simulink model "ModeleRobot"  (Simulink 7.4)
settings: Solver=FixedStepDiscrete  StartTime=0.0  StopTime=Inf  FixedStep=Te  RelTol=1e-3
values from neighbouring files (symbols this model uses):
  EQUIPE_JAUNE = 0    [ModeleRobot_ini.m]
  EQUIPE_VERTE = 1    [ModeleRobot_ini.m]
  JUST_HOMOLO = 1    [ModeleRobot_ini.m]
  MAX_SPEED_SERVOS = 0    [ModeleRobot_ini.m]
  PI = pi    (= 3.14159265359)    [ModeleRobot_ini.m]
  SERVO_BRAS_D = 14    [ModeleRobot_ini.m]
  SERVO_BRAS_D_FERME = 5    [ModeleRobot_ini.m]
  SERVO_BRAS_D_OUVERT = 104    [ModeleRobot_ini.m]
  SERVO_BRAS_G = 15    [ModeleRobot_ini.m]
  SERVO_BRAS_G_FERME = 18    [ModeleRobot_ini.m]
  SERVO_BRAS_G_OUVERT = 62    [ModeleRobot_ini.m]
  SERVO_INCLINAISON = 13    [ModeleRobot_ini.m]
  SERVO_INCLINAISON_DROIT = 143    [ModeleRobot_ini.m]
  SERVO_INCLINAISON_PENCHE = 24    [ModeleRobot_ini.m]
  STT = 1    [ModeleRobot_ini.m]
  Te = 0.02    [ModeleRobot_ini.m]
undefined symbols (not defined in the file or in its folder): SERVO_BEQUILLE
libraries: simulink x10
settings Model: Creator=Admin  LastModifiedBy=PC
settings DataIOCC: LimitDataPoints=off  SaveFormat=StructureWithTime
settings OptimizationCC: UseIntDivNetSlope=on  PassReuseOutputArgsAs=Individual arguments  ZeroExternalMemoryAtStartup=off  ZeroInternalMemoryAtStartup=off  EfficientFloat2IntCast=on  OptimizeModelRefInitCode=on  LifeSpan=Inf
settings DebuggingCC: SaveWithParameterizedLinksMsg=none  SignalResolutionControl=TryResolveAllWithWarning  MultiTaskDSMMsg=warning  MultiTaskCondExecSysMsg=none
settings HardwareCC: ProdIntDivRoundTo=Zero  ProdEndianess=LittleEndian  ProdHWDeviceType=Generic->32-bit x86 compatible
settings SFSimCC: SFSimEnableDebug=off  SFSimOverflowDetection=off  SFSimEcho=off  SimIntegrity=off  SimBuildMode=sf_nonincremental_build
settings RTWCC: SystemTargetFile=ert.tlc  GenCodeOnly=on  GenerateMakefile=off  TemplateMakefile=ert_default_tmf  PostCodeGenCommand=packNGo(buildInfo);  Description=Real-Time Workshop Embedded Coder  ProcessScript=ert_make_rtw_hook  IncludeERTFirstTime=on  RTWCompilerOptimization=On  CheckMdlBeforeBuild=Warning
settings CodeAppCC: IgnoreCustomStorageClasses=off
settings ERTTargetCC: UtilityFuncGeneration=Shared location  MultiwordLength=2048  IncludeMdlTerminateFcn=off  SuppressErrorStatus=on  SupportNonFinite=off  ERTCustomFileTemplate=example_file_process.tlc  GlobalDataDefinition=InSourceFile  GlobalDataReference=InSourceFile  ConvertIfToSwitch=off

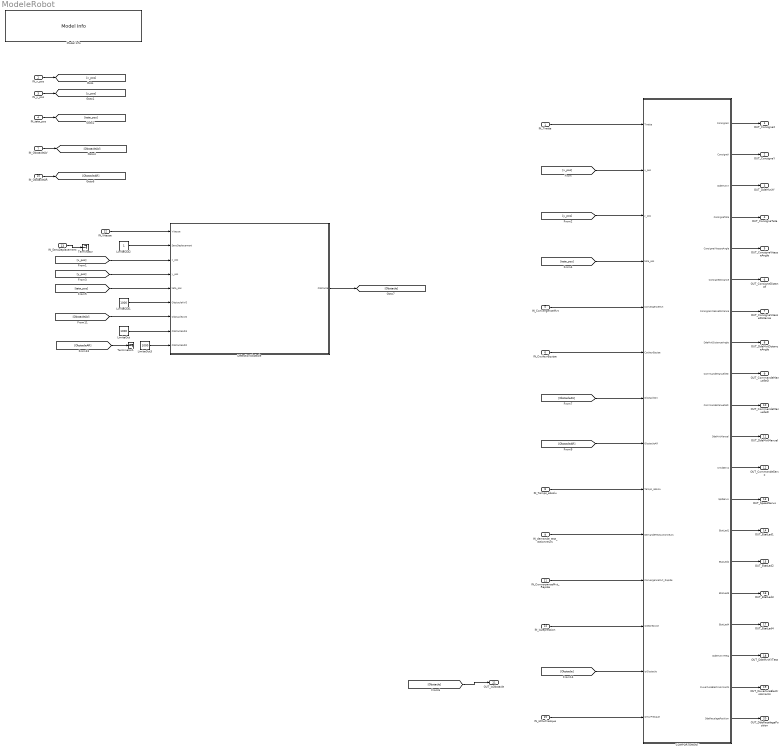
== system ModeleRobot ==
  IN_Tirette : Inport  OutDataType=sfix(16)  OutScaling=2^0
  IN_x_pos : Inport  Port=2  OutDataType=sfix(16)  OutScaling=2^0
  IN_y_pos : Inport  Port=3  OutDataType=sfix(16)  OutScaling=2^0
  IN_teta_pos : Inport  Port=4  OutDataType=sfix(16)  OutScaling=2^0
  IN_ConvergenceMvt : Inport  Port=5  OutDataType=sfix(16)  OutScaling=2^0
  IN_CouleurEquipe : Inport  Port=6  OutDataType=sfix(16)  OutScaling=2^0
  IN_ObstacleAV : Inport  Port=7  OutDataType=sfix(16)  OutScaling=2^0
  IN_Temps_absolu : Inport  Port=8  OutDataType=sfix(16)  OutScaling=2^0
  IN_demande_test_actionneurs : Inport  Port=9  OutDataType=sfix(16)  OutScaling=2^0
  IN_ObstacleAR : Inport  Port=10  OutDataType=sfix(16)  OutScaling=2^0
  IN_ConvergenceMvt_Rapide : Inport  Port=11  OutDataType=sfix(16)  OutScaling=2^0
  IN_Vitesse : Inport  Port=12  OutDataType=sfix(16)  OutScaling=2^0
  IN_SensDeplacement : Inport  Port=13  OutDataType=sfix(16)  OutScaling=2^0
  IN_isDepression : Inport  Port=14  OutDataType=sfix(16)  OutScaling=2^0
  IN_isMurFresque : Inport  Port=15  OutDataType=sfix(16)  OutScaling=2^0
  COMPORTEMENT : Stateflow chart
  DetectionObstacle : Subsystem
  LimiteOut : Constant  Value=1000  OutDataType=fixdt(1, 16)  OutScaling=2^0
  LimiteOut1 : Constant  Value=1000  OutDataType=fixdt(1, 16)  OutScaling=2^0
  LimiteOut2 : Constant  OutDataType=fixdt(1, 16)  OutScaling=2^0
  LimiteOut3 : Constant  Value=1000  OutDataType=fixdt(1, 16)  OutScaling=2^0
  Model Info : simulink/Model-Wide Utilities/Model Info  SystemSampleTime=-1  InitialBlockCM=None  BlockCM=None  Frame=on  DisplayStringWithTags=|  HorizontalTextAlignment=Left  LeftAlignmentValue=0.02  SourceBlockDiagram=ModeleRobot  TagMaxNumber=20
      | Description du comportement d'un robot
      | Objectif du robot :
  Terminator : Terminator
  Terminator1 : Terminator
  OUT_ConsigneX : Outport  OutDataType=sfix(16)  OutScaling=2^0
  OUT_ConsigneY : Outport  Port=2  OutDataType=sfix(16)  OutScaling=2^0
  OUT_DdeMvtXY : Outport  Port=3  OutDataType=sfix(16)  OutScaling=2^0
  OUT_ConsigneTeta : Outport  Port=4  OutDataType=sfix(16)  OutScaling=2^0
  OUT_ConsigneVitesseAngle : Outport  Port=5  OutDataType=sfix(16)  OutScaling=2^0
  OUT_ConsigneDistance : Outport  Port=6  OutDataType=sfix(16)  OutScaling=2^0
  OUT_ConsigneVitesseDistance : Outport  Port=7  OutDataType=sfix(16)  OutScaling=2^0
  OUT_DdeMvtDistanceAngle : Outport  Port=8  OutDataType=sfix(16)  OutScaling=2^0
  OUT_CommandeManuelleG : Outport  Port=9  OutDataType=sfix(16)  OutScaling=2^0
  OUT_CommandeManuelleD : Outport  Port=10  OutDataType=sfix(16)  OutScaling=2^0
  OUT_DdeMvtManuel : Outport  Port=11  OutDataType=sfix(16)  OutScaling=2^0
  OUT_CommandeServo : Outport  Port=12  OutDataType=sfix(16)  OutScaling=2^0
  OUT_SpeedServo : Outport  Port=13  OutDataType=sfix(16)  OutScaling=2^0
  OUT_EtatLed1 : Outport  Port=14  OutDataType=sfix(16)  OutScaling=2^0
  OUT_EtatLed2 : Outport  Port=15  OutDataType=sfix(16)  OutScaling=2^0
  OUT_EtatLed3 : Outport  Port=16  OutDataType=sfix(16)  OutScaling=2^0
  OUT_EtatLed4 : Outport  Port=17  OutDataType=sfix(16)  OutScaling=2^0
  OUT_DdeMvtXYTeta : Outport  Port=18  OutDataType=sfix(16)  OutScaling=2^0
  OUT_OuvertureElectroAimants : Outport  Port=19  OutDataType=sfix(16)  OutScaling=2^0
  OUT_DdeRecalagePosition : Outport  Port=20  OutDataType=sfix(16)  OutScaling=2^0
  OUT_isObstacle : Outport  Port=21  OutDataType=sfix(16)  OutScaling=2^0
  wires:
  COMPORTEMENT/1(ConsigneX) -> OUT_ConsigneX/1
  COMPORTEMENT/2(ConsigneY) -> OUT_ConsigneY/1
  IN_Temps_absolu/1 -> COMPORTEMENT/9(Temps_absolu)
  IN_ConvergenceMvt/1 -> COMPORTEMENT/5(ConvergenceMvt)
  IN_CouleurEquipe/1 -> COMPORTEMENT/6(CouleurEquipe)
  IN_Tirette/1 -> COMPORTEMENT/1(Tirette)
  IN_demande_test_actionneurs/1 -> COMPORTEMENT/10(DemandeTestActionneurs)
  COMPORTEMENT/3(DdeMvtXY) -> OUT_DdeMvtXY/1
  COMPORTEMENT/4(ConsigneTeta) -> OUT_ConsigneTeta/1
  COMPORTEMENT/5(ConsigneVitesseAngle) -> OUT_ConsigneVitesseAngle/1
  COMPORTEMENT/6(ConsigneDistance) -> OUT_ConsigneDistance/1
  COMPORTEMENT/7(ConsigneVitesseDistance) -> OUT_ConsigneVitesseDistance/1
  COMPORTEMENT/8(DdeMvtDistanceAngle) -> OUT_DdeMvtDistanceAngle/1
  COMPORTEMENT/9(CommandeManuelleG) -> OUT_CommandeManuelleG/1
  COMPORTEMENT/10(CommandeManuelleD) -> OUT_CommandeManuelleD/1
  COMPORTEMENT/11(DdeMvtManuel) -> OUT_DdeMvtManuel/1
  COMPORTEMENT/12(CmdServo) -> OUT_CommandeServo/1
  COMPORTEMENT/13(SpdServo) -> OUT_SpeedServo/1
  COMPORTEMENT/14(EtatLed1) -> OUT_EtatLed1/1
  COMPORTEMENT/15(EtatLed2) -> OUT_EtatLed2/1
  COMPORTEMENT/16(EtatLed3) -> OUT_EtatLed3/1
  COMPORTEMENT/17(EtatLed4) -> OUT_EtatLed4/1
  [x_pos] -> COMPORTEMENT/2(x_pos)
  [y_pos] -> COMPORTEMENT/3(y_pos)
  [teta_pos] -> COMPORTEMENT/4(teta_pos)
  IN_Vitesse/1 -> DetectionObstacle/1(Vitesse)
  [x_pos] -> DetectionObstacle/3(x_pos)
  [y_pos] -> DetectionObstacle/4(y_pos)
  [teta_pos] -> DetectionObstacle/5(teta_pos)
  IN_x_pos/1 -> [x_pos]
  IN_y_pos/1 -> [y_pos]
  IN_teta_pos/1 -> [teta_pos]
  COMPORTEMENT/18(DdeMvtXYTeta) -> OUT_DdeMvtXYTeta/1
  IN_ObstacleAV/1 -> [ObstacleAV]
  IN_ObstacleAR/1 -> [ObstacleAR]
  [ObstacleAV] -> COMPORTEMENT/7(ObstacleAV)
  [ObstacleAR] -> COMPORTEMENT/8(ObstacleAR)
  [ObstacleAV] -> DetectionObstacle/7(ObstacleAVD)
  DetectionObstacle/1(Obstacle) -> [Obstacle]
  [Obstacle] -> COMPORTEMENT/13(isObstacle)
  COMPORTEMENT/19(OuvertureElectroAimants) -> OUT_OuvertureElectroAimants/1
  IN_ConvergenceMvt_Rapide/1 -> COMPORTEMENT/11(ConvergenceMvt_Rapide)
  IN_isDepression/1 -> COMPORTEMENT/12(isDepression)
  LimiteOut1/1 -> DetectionObstacle/6(ObstacleAVG)
  LimiteOut/1 -> DetectionObstacle/8(ObstacleARG)
  COMPORTEMENT/20(DdeRecalagePosition) -> OUT_DdeRecalagePosition/1
  [Obstacle] -> OUT_isObstacle/1
  IN_isMurFresque/1 -> COMPORTEMENT/14(isMurFresque)
  LimiteOut2/1 -> DetectionObstacle/2(SensDeplacement)
  IN_SensDeplacement/1 -> Terminator/1
  [ObstacleAR] -> Terminator1/1
  LimiteOut3/1 -> DetectionObstacle/9(ObstacleARD)

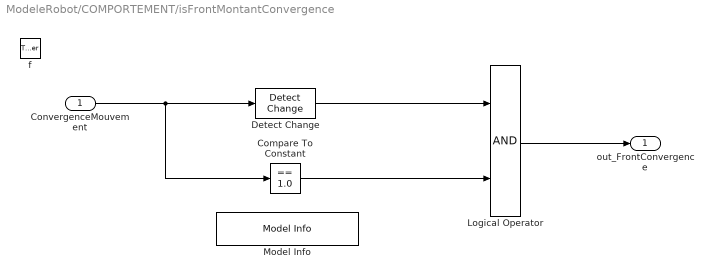
== system ModeleRobot/COMPORTEMENT/isFrontMontantConvergence ==
  ConvergenceMouvement : Inport
  f : TriggerPort  TriggerType=function-call
      settings: CopyFcn=set_param(gcbh,'PreDeleteFcn','')  PreDeleteFcn=Stateflow.SLINSF.SimulinkMan.unsafePredeleteFcn
  Compare To Constant : simulink/Logic and Bit Operations/Compare To Constant  SystemSampleTime=-1  relop===  const=1.0  LogicOutDataTypeMode=uint8
  Detect Change : simulink/Logic and Bit Operations/Detect Change  SystemSampleTime=-1  vinit=0
  Logical Operator : Logic  AllPortsSameDT=off  OutDataTypeMode=boolean  LogicDataType=fixdt(0, 8)  OutDataTypeStr=boolean
  Model Info : simulink/Model-Wide Utilities/Model Info  SystemSampleTime=-1  InitialBlockCM=None  BlockCM=None  Frame=off  DisplayStringWithTags="\"1\" = mouvement terminé"  HorizontalTextAlignment=Center  LeftAlignmentValue=0.5  SourceBlockDiagram=ModeleRobot  TagMaxNumber=20
  out_FrontConvergence : Outport
  wires:
  ConvergenceMouvement/1 -> Detect Change/1, Compare To Constant/1
  Detect Change/1 -> Logical Operator/1
  Compare To Constant/1 -> Logical Operator/2
  Logical Operator/1 -> out_FrontConvergence/1

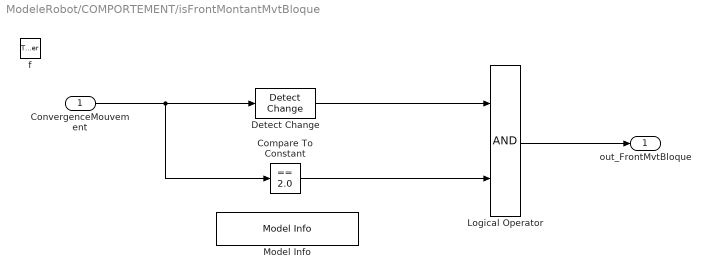
== system ModeleRobot/COMPORTEMENT/isFrontMontantMvtBloque ==
  ConvergenceMouvement : Inport
  f : TriggerPort  TriggerType=function-call
      settings: CopyFcn=set_param(gcbh,'PreDeleteFcn','')  PreDeleteFcn=Stateflow.SLINSF.SimulinkMan.unsafePredeleteFcn
  Compare To Constant : simulink/Logic and Bit Operations/Compare To Constant  SystemSampleTime=-1  relop===  const=2.0  LogicOutDataTypeMode=uint8
  Detect Change : simulink/Logic and Bit Operations/Detect Change  SystemSampleTime=-1  vinit=0
  Logical Operator : Logic  AllPortsSameDT=off  OutDataTypeMode=boolean  LogicDataType=fixdt(0, 8)  OutDataTypeStr=boolean
  Model Info : simulink/Model-Wide Utilities/Model Info  SystemSampleTime=-1  InitialBlockCM=None  BlockCM=None  Frame=off  DisplayStringWithTags="\"2\" = mouvement bloqué"  HorizontalTextAlignment=Center  LeftAlignmentValue=0.5  SourceBlockDiagram=ModeleRobot  TagMaxNumber=20
  out_FrontMvtBloque : Outport
  wires:
  ConvergenceMouvement/1 -> Detect Change/1, Compare To Constant/1
  Detect Change/1 -> Logical Operator/1
  Compare To Constant/1 -> Logical Operator/2
  Logical Operator/1 -> out_FrontMvtBloque/1

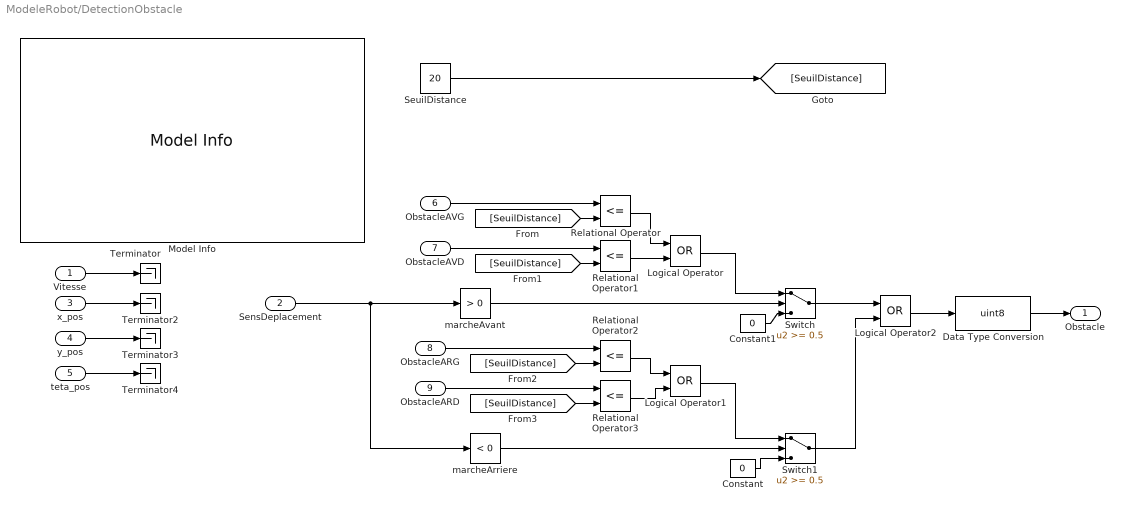
== system ModeleRobot/DetectionObstacle ==
  Vitesse : Inport  OutDataType=fixdt(1, 16)  OutScaling=2^0
  SensDeplacement : Inport  Port=2  OutDataType=fixdt(1, 16)  OutScaling=2^0
  x_pos : Inport  Port=3  OutDataType=fixdt(1, 16)  OutScaling=2^0
  y_pos : Inport  Port=4  OutDataType=fixdt(1, 16)  OutScaling=2^0
  teta_pos : Inport  Port=5  OutDataType=fixdt(1, 16)  OutScaling=2^0
  ObstacleAVG : Inport  Port=6  OutDataType=fixdt(1, 16)  OutScaling=2^0
  ObstacleAVD : Inport  Port=7  OutDataType=fixdt(1, 16)  OutScaling=2^0
  ObstacleARG : Inport  Port=8  OutDataType=fixdt(1, 16)  OutScaling=2^0
  ObstacleARD : Inport  Port=9  OutDataType=fixdt(1, 16)  OutScaling=2^0
  Constant : Constant  Value=0  OutDataType=fixdt(1, 16)  OutScaling=2^0
  Constant1 : Constant  Value=0  OutDataType=fixdt(1, 16)  OutScaling=2^0
  Data Type Conversion : DataTypeConversion  OutDataTypeMode=uint8  OutDataType=fixdt(1, 16)  OutScaling=2^0  OutDataTypeStr=uint8
  Logical Operator : Logic  Operator=OR  AllPortsSameDT=off  OutDataTypeMode=boolean  LogicDataType=fixdt(0, 8)  OutDataTypeStr=boolean
  Logical Operator1 : Logic  Operator=OR  AllPortsSameDT=off  OutDataTypeMode=boolean  LogicDataType=fixdt(0, 8)  OutDataTypeStr=boolean
  Logical Operator2 : Logic  Operator=OR  AllPortsSameDT=off  OutDataTypeMode=boolean  LogicDataType=fixdt(0, 8)  OutDataTypeStr=boolean
  Model Info : simulink/Model-Wide Utilities/Model Info  SystemSampleTime=-1  InitialBlockCM=None  BlockCM=None  Frame=on  DisplayStringWithTags=|  HorizontalTextAlignment=Left  LeftAlignmentValue=0.02  SourceBlockDiagram=ModeleRobot  TagMaxNumber=20
      | Description de la détection d'obstacle
      | Obstacle :
      | Suivant le sens de la marche on active la détection par capteur US (donne une distance). Fonction d'un seuil de distance on tilte sur la présence d'un obstacle. On synthétise les détection arrière et avant pour avoir une seule info de détection d'obstacle pour la stratégie.
      | 
      | TODO:
      | * faire varier le seuil de détection en fonction de la vitesse.
      | * utiliser la position et l'orientation du robot pour discriminer un élément du terrain.
  Relational Operator{,1..3} (4 alike) : RelationalOperator  Operator=<=  LogicOutDataTypeMode=boolean  LogicDataType=fixdt(0, 8)  OutDataTypeStr=boolean
  SeuilDistance : Constant  Value=20  OutDataType=fixdt(1, 16)  OutScaling=2^0
  Switch : Switch  Threshold=0.5  OutDataType=fixdt(1, 16)  OutScaling=2^0
  Switch1 : Switch  Threshold=0.5  OutDataType=fixdt(1, 16)  OutScaling=2^0
  Terminator{,2..4} (4 alike) : Terminator
  marcheArriere : simulink/Logic and Bit Operations/Compare To Zero  SystemSampleTime=-1  relop=<  LogicOutDataTypeMode=uint8
  marcheAvant : simulink/Logic and Bit Operations/Compare To Zero  SystemSampleTime=-1  relop=>  LogicOutDataTypeMode=uint8
  Obstacle : Outport  OutDataType=fixdt(1, 16)  OutScaling=2^0
  wires:
  Vitesse/1 -> Terminator/1
  SensDeplacement/1 -> marcheAvant/1, marcheArriere/1
  x_pos/1 -> Terminator2/1
  y_pos/1 -> Terminator3/1
  teta_pos/1 -> Terminator4/1
  marcheAvant/1 -> Switch/2
  Relational Operator1/1 -> Logical Operator/2
  ObstacleARD/1 -> Relational Operator3/1
  marcheArriere/1 -> Switch1/2
  Relational Operator2/1 -> Logical Operator1/1
  Constant/1 -> Switch1/3
  Switch/1 -> Logical Operator2/1
  Switch1/1 -> Logical Operator2/2
  Logical Operator2/1 -> Data Type Conversion/1
  Relational Operator/1 -> Logical Operator/1
  ObstacleAVG/1 -> Relational Operator/1
  ObstacleAVD/1 -> Relational Operator1/1
  ObstacleARG/1 -> Relational Operator2/1
  SeuilDistance/1 -> [SeuilDistance]
  [SeuilDistance] -> Relational Operator/2
  [SeuilDistance] -> Relational Operator3/2
  [SeuilDistance] -> Relational Operator2/2
  [SeuilDistance] -> Relational Operator1/2
  Constant1/1 -> Switch/3
  Relational Operator3/1 -> Logical Operator1/2
  Logical Operator1/1 -> Switch1/1
  Logical Operator/1 -> Switch/1
  Data Type Conversion/1 -> Obstacle/1

== stateflow chart COMPORTEMENT ==
  state COMPORTEMENT_ROBOT [parallel]
    settings: executionOrder=1
    state ATTENTE_TIRETTE/
      state ACTIONNEURS_REPOS/ [parallel]
        settings: executionOrder=1
        state REPOS_SERVOS/
          entry :
          Mouvement_Manuel(0, 0);
          setServoSpeed(SERVO_BRAS_G, MAX_SPEED_SERVOS);
          setServoSpeed(SERVO_BRAS_D, MAX_SPEED_SERVOS);
          setServoSpeed(SERVO_INCLINAISON, MAX_SPEED_SERVOS);
          setServo(SERVO_BRAS_G, SERVO_BRAS_G_FERME);
          setServo(SERVO_BRAS_D, SERVO_BRAS_D_FERME);
          setServo(SERVO_INCLINAISON, SERVO_INCLINAISON_DROIT);
          TempoInit=0;
          during:
          TempoInit++;
        state FIN_REPOS_ACTIONNEUR/
          entry:
          setServo(SERVO_BRAS_G, SERVO_BRAS_G_FERME);
          setServo(SERVO_BRAS_D, SERVO_BRAS_D_FERME);
          setServo(SERVO_INCLINAISON, SERVO_INCLINAISON_DROIT);
          TempoInit=0;
        (default) -> REPOS_SERVOS
        REPOS_SERVOS -> FIN_REPOS_ACTIONNEUR : [TempoInit>(2/Te)]
      state CHOIX_EQUIPE/ [parallel]
        exit :
        CouleurEquipe_memo = CouleurEquipe;
        settings: executionOrder=2
        state EQUIPE_2/
          entry :
          EtatLed1 = 0;
          EtatLed2 = 1;
          invMouv=1;
        state EQUIPE_1/
          entry :
          EtatLed1 = 1;
          EtatLed2 = 0;
          invMouv=-1;
        (default) -> EQUIPE_1
        EQUIPE_1 -> EQUIPE_2 : [CouleurEquipe == EQUIPE_JAUNE]
        EQUIPE_2 -> EQUIPE_1 : [CouleurEquipe == EQUIPE_VERTE]
      state RECALAGE/ [parallel]
        //TODO: a faire si on veut respecter les coordonnees reelles du terrain
        settings: executionOrder=3
        state INIT/
          entry :
          x_offset = 0;
          y_offset=0;
          theta_offset=0;
        (default) -> COMPORTEMENT_ROBOT.ATTENTE_TIRETTE.RECALAGE.INIT
      state TESTS_ACTIONNEUR/ [parallel]
        entry:
        TempoTestActionneurs=0;
        during :
        TempoTestActionneurs++;
        settings: executionOrder=4
        state TEST_ACT_3/
          entry:
          TempoTestActionneurs = 0;
          setServo(SERVO_BRAS_G, SERVO_BRAS_G_OUVERT);
          setServo(SERVO_BRAS_D, SERVO_BRAS_D_FERME);
          setServo(SERVO_INCLINAISON, SERVO_INCLINAISON_DROIT);
        state TEST_ACT_FIN/
          entry:
          TempoTestActionneurs = 0;
          test_actionneurs_en_cours=0;
        state TEST_ACT_6/
          entry:
          TempoTestActionneurs = 0;
          setServo(SERVO_BRAS_G, SERVO_BRAS_G_FERME);
          setServo(SERVO_BRAS_D, SERVO_BRAS_D_FERME);
          setServo(SERVO_INCLINAISON, SERVO_INCLINAISON_DROIT);
        state INIT/
          entry:
          test_actionneurs_en_cours=0;
        state TEST_ACT_4/
          entry:
          TempoTestActionneurs = 0;
          setServo(SERVO_BRAS_G, SERVO_BRAS_G_FERME);
          setServo(SERVO_BRAS_D, SERVO_BRAS_D_OUVERT);
          setServo(SERVO_INCLINAISON, SERVO_INCLINAISON_DROIT);
        state TEST_ACT_5/
          entry:
          TempoTestActionneurs = 0;
          setServo(SERVO_BRAS_G, SERVO_BRAS_G_FERME);
          setServo(SERVO_BRAS_D, SERVO_BRAS_D_FERME);
          setServo(SERVO_INCLINAISON, SERVO_INCLINAISON_PENCHE);
        state INIT1/
          entry:
          test_actionneurs_en_cours=1;
          TempoTestActionneurs = 0;
        TEST_ACT_6 -> TEST_ACT_FIN : [TempoTestActionneurs > (2/Te)]
        (junction 78) -> INIT1 : [DemandeTestActionneurs != 0]
        TEST_ACT_5 -> TEST_ACT_6 : [TempoTestActionneurs > (2/Te)]
        TEST_ACT_FIN -> (junction 78)
        (default) -> COMPORTEMENT_ROBOT.ATTENTE_TIRETTE.TESTS_ACTIONNEUR.INIT
        COMPORTEMENT_ROBOT.ATTENTE_TIRETTE.TESTS_ACTIONNEUR.INIT -> (junction 78)
        TEST_ACT_4 -> TEST_ACT_5 : [TempoTestActionneurs > (2/Te)]
        TEST_ACT_3 -> TEST_ACT_4 : [TempoTestActionneurs > (2/Te)]
        INIT1 -> TEST_ACT_3 : [TempoTestActionneurs > (1/Te)]
      state TESTS_CAPTEURS/ [parallel]
        during:
        //CommandeLEDS(1,1, 1,1);
        settings: executionOrder=5
    state FIN_MATCH/
      state FIN_MATCH_01/
        entry:
        Mouvement_Manuel(0, 0);
        setServo(SERVO_BRAS_G, SERVO_BRAS_G_FERME);
        setServo(SERVO_BRAS_D, SERVO_BRAS_D_FERME);
        setServo(SERVO_INCLINAISON, SERVO_INCLINAISON_DROIT);
        CommandeLEDS(1, 1, 1, 1);
        TempoImage=0;
        during:
        TempoImage++;
      state FIN_MATCH_02/
        entry:
        //chenillard de led
        CommandeLEDS(1, 0, 0, 0);
        TempoImage=0;
        during:
        TempoImage++;
      state FIN_MATCH_04/
        entry:
        //chenillard de led
        CommandeLEDS(0, 0, 1, 0);
        TempoImage=0;
        during:
        TempoImage++;
      state FIN_MATCH_03/
        entry:
        //chenillard de led
        CommandeLEDS(0, 1, 0, 0);
        TempoImage=0;
        during:
        TempoImage++;
      state FIN_MATCH_05/
        entry:
        //chenillard de led
        CommandeLEDS(0, 0, 0, 1);
        TempoImage=0;
        during:
        TempoImage++;
      FIN_MATCH_01 -> FIN_MATCH_02 : [TempoImage>(3/Te)]
      (default) -> FIN_MATCH_01
      FIN_MATCH_03 -> FIN_MATCH_04 : [(TempoImage>(1/Te))]
      FIN_MATCH_04 -> FIN_MATCH_05 : [(TempoImage>(1/Te))]
      FIN_MATCH_05 -> FIN_MATCH_02 : [(TempoImage>(1/Te))]
      FIN_MATCH_02 -> FIN_MATCH_03 : [(TempoImage>(1/Te))]
    state MATCH/
      state STRATEGIE/ [parallel]
        settings: executionOrder=2
        state STRATEGIE1
          //during:
          //CommandeLEDS_RVBO(ObstacleARG,ObstacleARD, ObstacleAVG,ObstacleAVD);
          (history)
          state INIT_STRATEGIE/
            entry :
            ConsigneVitesseAngle = 3; // [rad/sec]
            ConsigneVitesseDistance = 80; //[cm/sec]
            inhibeObstacle=0;
            finHomologation=0;
          state GOTO_BAS_DES_MARCHES/
            entry:
            Tempo=0;
            DistanceParcourue=0;DistanceParcourue2=0;
            x_old=0;y_old=0;   x_old2=0;y_old2=0;
            x_temp=0;y_temp=0;
            inhibeObstacle=0;
            Etape_GotoMarche=1;
            during:
            Tempo++;
            (history)
            state HOMOLO_FIN/
              entry:
              // Fin - en cours de debuggage on ne sort pour l'instant pas de l'homologation
              finHomologation=0;
              Etape_GotoMarche=0;
            state ACTION_04
              entry:
              Mouvement_Manuel(0, 0);
            state ACTION_03
              entry:
              Tempo=0;
              Mouvement_Manuel(0, 0);
            state ACTION_01
              entry:
              Tempo=0;
              Mouvement_Manuel(100, 100);
            state ACTION_02
              entry:
              Tempo=0;
              Mouvement_Manuel(100, 100);
            state ACTION_05
              entry:
              Tempo=0;
              Mouvement_Manuel(100, 0);
            state ACTION_06
              entry:
              Tempo=0;
              Mouvement_Manuel(0, 100);
            ACTION_04 -> HOMOLO_FIN
            (default) -> COMPORTEMENT_ROBOT.MATCH.STRATEGIE.STRATEGIE1.GOTO_BAS_DES_MARCHES.ACTION_01
            ACTION_03 -> ACTION_04 : [Tempo>(2.3/Te)]
            COMPORTEMENT_ROBOT.MATCH.STRATEGIE.STRATEGIE1.GOTO_BAS_DES_MARCHES.ACTION_01 -> (junction 91) : [Tempo>(9.3/Te)]
            ACTION_02 -> ACTION_03 : [Tempo>(5/Te)]
            (junction 91) -> ACTION_05 [order 2]
            (junction 91) -> ACTION_06 [order 1] : [CouleurEquipe_memo == EQUIPE_VERTE]
            ACTION_05 -> (junction 92)
            ACTION_06 -> (junction 92)
            (junction 92) -> ACTION_02 : [Tempo>(2.65/Te)]
          state MONTE_MARCHE/
            entry:
            Tempo=0;
            inhibeObstacle=1;  // Pas de détection d'obostacle pendant la montée des marches
            during:
            Tempo++;
            (history)
            state ACTION_01
              entry:
              Tempo=0;
              Mouvement_Manuel(0, 0);
            (default) -> COMPORTEMENT_ROBOT.MATCH.STRATEGIE.STRATEGIE1.MONTE_MARCHE.ACTION_01
          (default) -> INIT_STRATEGIE
          INIT_STRATEGIE -> GOTO_BAS_DES_MARCHES : [DureeMatch > (0.04/Te)]
          GOTO_BAS_DES_MARCHES -> MONTE_MARCHE : [Etape_GotoMarche==0]
        state EVITEMENT/
          entry :
          EvitementEnCours  = 1;
          //Dans le cas d'un mouvement distance on calcule la distance parcourue pour repartir
          //avec une consigne adapte
          DistanceParcourue=sqrt((x_pos-x_old)^2+(y_pos-y_old)^2);
          local_Tempo=0;
          during :
          local_Tempo++;
          state DETECT_OBSTACLE/
            entry :
            local_Tempo = 0;
            //Mouvement_ArretBrutal(); // Arrête tout pendant un instant mais bug
            Mouvement_Manuel(0,0);
            CommandeLEDS(1,0,0,0);
          state DETECT_OBSTACLE1/
            entry :
            ConsigneVitesseAngle = 3; // [rad/sec]
            ConsigneVitesseDistance = 40; //[cm/sec]
            EvitementEnCours = 0;
          (default) -> DETECT_OBSTACLE
          DETECT_OBSTACLE -> DETECT_OBSTACLE1 : [local_Tempo > (2/Te)]
        STRATEGIE1 -> EVITEMENT : [(isObstacle==1) && (inhibeObstacle==0)]
        (default) -> STRATEGIE1
        EVITEMENT -> STRATEGIE1 : [(EvitementEnCours==0)]
      state CLOCK [parallel]
        during : DureeMatch++
        settings: executionOrder=1
    (default) -> ATTENTE_TIRETTE
    MATCH -> FIN_MATCH : [DureeMatch > (90/Te)]
    ATTENTE_TIRETTE -> MATCH : [Tirette != 0]
  state ret = isFinMouvement(timeout) [function]
    (junction 71) -> (junction 72) : { ret = (CompteurTimeoutMvt > timeout) || (isFrontMontantConvergence(ConvergenceMvt));}
    (default) -> (junction 71) : { CompteurTimeoutMvt++}
  state FONCTIONS_GLOBALES_DEPLACEMENT_ROBOT [parallel]
    settings: executionOrder=2
  state Mouvement_Manuel(motG, motD) [function]
    (default) -> (junction 74) : {  DdeMvtManuel = DdeMvtManuel+1;...
        |    CommandeManuelleG = motG;...
        |    CommandeManuelleD = motD;...
        | }
  state FONCTIONS_GLOBALES_COMMANDE_LEDS [parallel]
    settings: executionOrder=5
  state FONCTIONS_GLOBALES_DETECTION_OBSTACLES [parallel]
    settings: executionOrder=4
  state ret = isFinMouvementRapide(timeout) [function]
    (junction 84) -> (junction 83) : { ret = (CompteurTimeoutMvt > timeout) || (isFrontMontantConvergence(ConvergenceMvt_Rapide));}
    (default) -> (junction 84) : { CompteurTimeoutMvt++}
  state FONCTIONS_GLOBALES_COMMANDE_SERVOS [parallel]
    settings: executionOrder=3
  state Mouvement_DistanceAngle(dist, teta_rad) [function]
    (default) -> (junction 73) : {  DdeMvtDistanceAngle++;...
        |    ConsigneDistance = dist;...
        |    ConsigneTeta = teta_rad;...
        |    % Modulo de l'angle fait dans le StrategieMatlab.c
        |    CompteurTimeoutMvt = 0;...
        | }
  state Mouvement_DistanceVitesse(dist, vitesse) [function]
    (default) -> (junction 86) : {  DdeMvtDistanceAngle++;...
        |    ConsigneDistance = dist;...
        |    ConsigneVitesseDistance = vitesse;...
        |    % ConsigneTeta reste inchangé.
        |    CompteurTimeoutMvt = 0;...
        | }
  state out_FrontConvergence  = isFrontMontantConvergence(ConvergenceMouvement) [function]
  state out_FrontMvtBloque  = isFrontMontantMvtBloque(ConvergenceMouvement) [function]
  state Mouvement_Angle(teta_rad) [function]
    (default) -> (junction 75) : {  DdeMvtDistanceAngle++;...
        |    ConsigneDistance = 0;...
        |    ConsigneTeta = teta_rad;...
        |    CompteurTimeoutMvt = 0;...
        | }
  state Mouvement_Distance(dist) [function]
    (default) -> (junction 76) : {  DdeMvtDistanceAngle++;...
        |    ConsigneDistance = dist;...
        |    % ConsigneTeta reste inchangé.
        |    CompteurTimeoutMvt = 0;...
        | }
  state CommandeLEDS(L1, L2, L3, L4) [function]
    (default) -> (junction 77) : {   EtatLed1 = L1;...
        |     EtatLed2 = L2;...
        |     EtatLed3 = L3;...
        |     EtatLed4 = L4;...
        | }
  state FONCTIONS_GLOBALES_DIVERS [parallel]
    settings: executionOrder=6
  state Mouvement_XY(x, y) [function]
    (default) -> (junction 80) : {  DdeMvtXY++;...
        |    ConsigneX = x;...
        |    ConsigneY = y;...
        |    CompteurTimeoutMvt = 0;...
        | }
  state ret = isMouvementBloque [function]
    (default) -> (junction 89) : { ret =(isFrontMontantMvtBloque(ConvergenceMvt));}
  state Mouvement_ArretBrutal [function]
    (default) -> (junction 88) : { ConsigneVitesseDistance=0;...
        | ConsigneVitesseAngle=0;}
  state RecalagePosition_XYTeta(x, y, teta) [function]
    (default) -> (junction 70) : {  DdeRecalagePosition++;...
        |    ConsigneX = x;...
        |    ConsigneY = y;...
        |    ConsigneTeta = teta
        | }
  state FONCTIONS_RECalAGE_POSITION [parallel]
    settings: executionOrder=7
  state setServoSpeed(idServo,vit) [function]
    (default) -> (junction 82) : {  SpdServo[idServo-1] = vit;
        |  }
  state Mouvement_XYTeta(x, y,teta_rad) [function]
    (default) -> (junction 85) : {  DdeMvtXYTeta++;...
        |    ConsigneX = x;...
        |    ConsigneY = y;...
        |    ConsigneTeta=teta_rad;...
        |    CompteurTimeoutMvt = 0;...
        | }
  state Mouvement_AngleVitesse(teta_rad, vitesse) [function]
    (default) -> (junction 79) : {  DdeMvtDistanceAngle++;...
        |    ConsigneDistance = 0;...
        |    ConsigneTeta = teta_rad;...
        |    ConsigneVitesseAngle = vitesse;...
        |    CompteurTimeoutMvt = 0;...
        | }
  state setServo(idServo,pos) [function]
    (default) -> (junction 90) : {  CmdServo[idServo-1] = pos;
        |  }
  data: ret function_output double; timeout function_input double; motG function_input double; motD function_input double; ret function_output double; timeout function_input double; dist function_input double; teta_rad function_input double; dist function_input double; vitesse function_input double; out_FrontConvergence function_output double; ConvergenceMouvement function_input double; out_FrontMvtBloque function_output double; ConvergenceMouvement function_input double; teta_rad function_input double; dist function_input double; L1 function_input double; L2 function_input double; L3 function_input double; L4 function_input double; x function_input double; y function_input double; ret function_output double; x function_input double; y function_input double; teta function_input double; idServo function_input double; vit function_input double; x function_input double; y function_input double; teta_rad function_input double; teta_rad function_input double; vitesse function_input double; idServo function_input double; pos function_input double; Tirette input double; x_pos input double; y_pos input double; teta_pos input double; ConvergenceMvt input double; CouleurEquipe input double; ObstacleAV input double; ObstacleAR input double; Temps_absolu input double; ConsigneX output double; ConsigneY output double; DdeMvtXY output double; ConsigneTeta output double; ConsigneVitesseAngle output double; ConsigneDistance output double; ConsigneVitesseDistance output double; DdeMvtDistanceAngle output double; CommandeManuelleG output double; CommandeManuelleD output double; DdeMvtManuel output double; CmdServo output double size=20 =0; SpdServo output double size=20; DureeMatch local double; Te parameter double; EtatLed1 output double; EtatLed2 output double; EtatLed3 output double; EtatLed4 output double; CouleurEquipe_memo local double; EQUIPE_JAUNE parameter double; CompteurTimeoutMvt local double; TetaPos local double; invMouv local double; finHomologation local double; PI parameter double; Tempo local double; ConsigneAngle local double; STT parameter int8; TempoInit local double; JUST_HOMOLO parameter int8; TempoMot local double; theta_offset local double; x_offset local double; y_offset local double; DemandeTestActionneurs input uint8; test_actionneurs_en_cours local double; EQUIPE_VERTE parameter double; TempoTestActionneurs local double; MAX_SPEED_SERVOS parameter double; SERVO_INCLINAISON_PENCHE parameter double; EvitementEnCours local double; x_pos_objectif local double; y_pos_objectif local double; DistanceParcourue local double; x_old local double; x_temp local double; y_old local double; y_temp local double; DistanceParcourue2 local double; x_old2 local double; y_old2 local double; DdeMvtXYTeta output double; ConvergenceMvt_Rapide input double; isDepression input uint8; isObstacle input uint8; inhibeObstacle local double; OuvertureElectroAimants output double =0; SERVO_INCLINAISON_DROIT parameter double; SERVO_INCLINAISON parameter double; DdeRecalagePosition output double; TempoImage local double; local_Tempo local double; isMurFresque input uint8; SERVO_BRAS_D parameter double; SERVO_BRAS_D_OUVERT parameter double; SERVO_BRAS_G_FERME parameter double; SERVO_BRAS_G_OUVERT parameter double; SERVO_BRAS_D_FERME parameter double; SERVO_BEQUILLE parameter double; SERVO_BRAS_G parameter double; Etape_GotoMarche local double
